simulink model "PM_fnc17_DevHarness_rate_limiter_r03"  (R2022a)
settings: Solver=FixedStepAuto  StartTime=0.0  StopTime=60  FixedStep=fixedsteprate_s  RelTol=1e-3
values from neighbouring files (symbols this model uses):
  fixedsteprate_s = rate_s    (= 0.01)    [PM_fnc1000_tc01_iter01_testsignal_builder.m]    (also in PM_fnc21_tc01_iter01_testsignal_builder.m; PM_fnc22_tc01_iter01_testsignal_builder.m)
settings Model: NumberOfSteps=2  Creator=306427  LastModifiedBy=306427

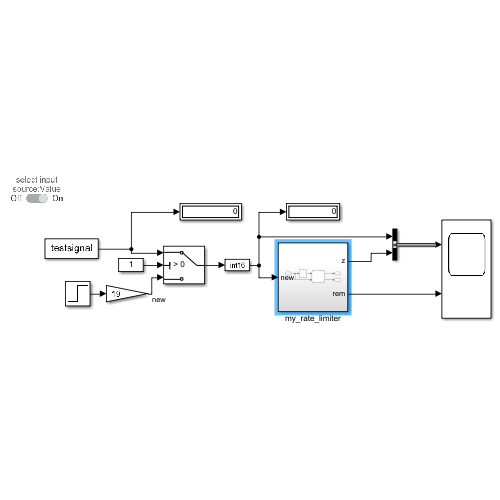
[thumbnail: Simulink's stored preview of the top-level diagram]
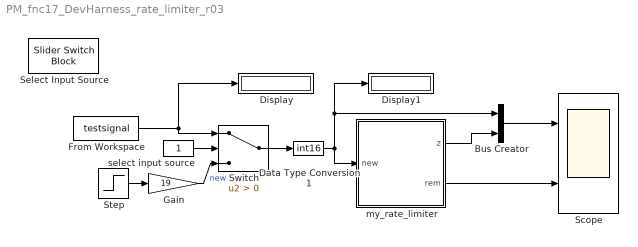
== system PM_fnc17_DevHarness_rate_limiter_r03 ==
  Bus Creator : BusCreator  Inputs=2
  Data Type Conversion1 : DataTypeConversion  OutDataTypeStr=int16  SaturateOnIntegerOverflow=off  RndMeth=Floor
  Display : Display
  Display1 : Display
  From Workspace : FromWorkspace  VariableName=testsignal  SampleTime=fixedsteprate_s
  Gain : Gain  Gain=19  OutDataTypeStr=int16  ParamDataTypeStr=Inherit: Same as input
  Scope : Scope  NumInputPorts=2
  Select Input Source : SliderSwitchBlock
      settings: Values={{'Off', 'On'}, [0 1]}
  Step : Step  SampleTime=fixedsteprate_s
  Switch : Switch  Criteria=u2 > Threshold  SaturateOnIntegerOverflow=off  InputSameDT=off
  my_rate_limiter : Subsystem
  select input source : Constant
  wires:
  Gain/1 -> Switch/3  "new"
  Bus Creator/1 -> Scope/1
  my_rate_limiter/1(z) -> Bus Creator/2
  my_rate_limiter/2(rem) -> Scope/2
  select input source/1 -> Switch/2
  From Workspace/1 -> Display/1, Switch/1
  Switch/1 -> Data Type Conversion1/1
  Data Type Conversion1/1 -> Bus Creator/1, Display1/1, my_rate_limiter/1(new)
  Step/1 -> Gain/1

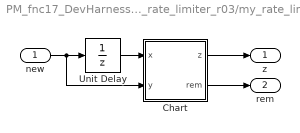
== system PM_fnc17_DevHarness_rate_limiter_r03/my_rate_limiter ==
  new : Inport
  Chart : Stateflow chart  TreatAsAtomicUnit=on
  Unit Delay : UnitDelay  SampleTime=-1  HasFrameUpgradeWarning=on
  z : Outport
  rem : Outport  Port=2
  wires:
  Unit Delay/1 -> Chart/1(x)
  new/1 -> Chart/2(y), Unit Delay/1
  Chart/1(z) -> z/1
  Chart/2(rem) -> rem/1

== stateflow chart PM_fnc17_DevHarness_rate_limiter_r03/my_rate_limiter/Chart ==
  note: Convention
      | next > prev is postive change/increase
      | next < prev is negative change/decrease
      |
      | This is a flat, single-state, looped-back state machine to eliminate any execution loop delays due to junctions and transitions from one state to another.
  note: if the difference is within the rate limit,
      | then just pass the "next" value
  state ZERO_REMAINDER
    prev = x;
    next = y;
    d_new = prev - prev_new;
    if d_new ~= 0  % prev_new has not caught up to prev
    prev = prev_new;
    elseif d_new == 0  % prev_new has caught up to prev
    prev = prev_new;
    end
    d = next - prev;
  (default) -> ZERO_REMAINDER : {remainder = 0;
      | prev_new = 0;}
  ZERO_REMAINDER -> ZERO_REMAINDER [order 1] : [-10 <= d && d < 0]/{...
      | z = next; rem = int16(0);}
  ZERO_REMAINDER -> ZERO_REMAINDER [order 4] : [0 < d && d <= 10]/{z = next; rem = int16(0);}
  ZERO_REMAINDER -> ZERO_REMAINDER [order 5] : [d == 0 && remainder > 0]/{...
      | temp = prev_new + 1;
      | prev_new = temp;
      | remainder = next - temp;
      | z = int16(temp);
      | rem = int16(remainder);}
  ZERO_REMAINDER -> ZERO_REMAINDER [order 6] : [d == 0 & remainder < 0]/{...
      | temp = prev_new - 1;
      | prev_new = temp;
      | remainder = next - z;
      | z = int16(temp);
      | rem = int16(remainder);}
  ZERO_REMAINDER -> ZERO_REMAINDER [order 2] : [d <= -10]/{...
      | temp = prev - 1;
      | prev_new = temp;
      | remainder = next - temp;
      | z = int16(temp);
      | rem = int16(remainder);}
  ZERO_REMAINDER -> ZERO_REMAINDER [order 3] : [10 <= d]/{...
      | temp = prev + 1;
      | prev_new = temp;
      | remainder = next - temp;
      | z = int16(temp);
      | rem = int16(remainder);}
  data: x input; prev local int16; y input; z output int16; next local int16; d local int16; prev_new local int16; rem output int16; remainder local int16; temp local int16; d_new local
